simulink model "ASM_Traffic_V2X_Complete_Model_2"  (R2019a)
settings: Solver=ode1  StartTime=SIM.tstart.v  StopTime=Inf  FixedStep=SIM.StepSize.v  RelTol=1e-3
PostLoadFcn:
  | if any(exist('dsrtsu_mdlpostloadfcn', 'file') ~= 0), dsrtsu_mdlpostloadfcn('Execute', bdroot); end
  | try, asm_mdl_postloadfcn(bdroot, 'UpdateModel', 2200); catch, disp(lasterr); end,
undefined symbols (not defined in the file): _SensorPnts_1, _SensorPnts_13, _SensorPnts_17, _SensorPnts_21, _SensorPnts_25, _SensorPnts_29, _SensorPnts_33, _SensorPnts_37, _SensorPnts_41, _SensorPnts_45, _SensorPnts_49, _SensorPnts_5, _SensorPnts_53, _SensorPnts_57, _SensorPnts_9, _to_, CPT, G5A, ITS, MDL, rad, s_to_rpm, SIM
libraries: simulink x169, ASM_VehicleDynamics_lib x126, ASM_Traffic_lib x83, ASM_Utils_lib x49, mdbs x45, ASM_Environment_lib x17, dspindex x12, dsaV2xLibraryAux x10, dsmpblib x6, dsaV2xAsn1Library x4, dsaV2xLibrary x4, ASM_BrakeHydraulics_lib x4
(part 35 of 36)

== system ASM_Traffic_V2X_Complete_Model_2/IO/I//O_Subsystem/Bus Configuration (1) - Out/Simulated ECUs/DrivekitCAN/Drivekit/RX/PDUs/STEERING_TORQUE_COMMAND/steering_torque_command ==
  steering_torque_command : Inport
  ISignal Value : Subsystem
  _steering_torque_command_ : BusSelector  OutputSignals=ISignal Value
  wires:
  steering_torque_command/1 -> _steering_torque_command_/1  "steering_torque_command"
  _steering_torque_command_/1 -> ISignal Value/1(ISignal Value)  "<ISignal Value>"

== system ASM_Traffic_V2X_Complete_Model_2/IO/I//O_Subsystem/Bus Configuration (1) - Out/Simulated ECUs/DrivekitCAN/Drivekit/RX/PDUs/THROTTLE_COMMAND/throttle_command_magic ==
  throttle_command_magic : Inport
  ISignal Value : Subsystem
  _throttle_command_magic_ : BusSelector  OutputSignals=ISignal Value
  wires:
  throttle_command_magic/1 -> _throttle_command_magic_/1  "throttle_command_magic"
  _throttle_command_magic_/1 -> ISignal Value/1(ISignal Value)  "<ISignal Value>"

== system ASM_Traffic_V2X_Complete_Model_2/IO/I//O_Subsystem/Bus Configuration (1) - Out/Simulated ECUs/DrivekitCAN/Drivekit/RX/PDUs/THROTTLE_COMMAND/throttle_pedal_command ==
  throttle_pedal_command : Inport
  ISignal Value : Subsystem
  _throttle_pedal_command_ : BusSelector  OutputSignals=ISignal Value
  wires:
  throttle_pedal_command/1 -> _throttle_pedal_command_/1  "throttle_pedal_command"
  _throttle_pedal_command_/1 -> ISignal Value/1(ISignal Value)  "<ISignal Value>"

== system ASM_Traffic_V2X_Complete_Model_2/IO/I//O_Subsystem/Bus Configuration (1) - Out/Simulated ECUs/DrivekitCAN/Drivekit/RX/PDUs/THROTTLE_DISABLE/throttle_disable_magic ==
  throttle_disable_magic : Inport
  ISignal Value : Subsystem
  _throttle_disable_magic_ : BusSelector  OutputSignals=ISignal Value
  wires:
  throttle_disable_magic/1 -> _throttle_disable_magic_/1  "throttle_disable_magic"
  _throttle_disable_magic_/1 -> ISignal Value/1(ISignal Value)  "<ISignal Value>"

== system ASM_Traffic_V2X_Complete_Model_2/IO/I//O_Subsystem/Bus Configuration (1) - Out/Simulated ECUs/DrivekitCAN/Drivekit/RX/PDUs/THROTTLE_ENABLE/throttle_enable_magic ==
  throttle_enable_magic : Inport
  ISignal Value : Subsystem
  _throttle_enable_magic_ : BusSelector  OutputSignals=ISignal Value
  wires:
  throttle_enable_magic/1 -> _throttle_enable_magic_/1  "throttle_enable_magic"
  _throttle_enable_magic_/1 -> ISignal Value/1(ISignal Value)  "<ISignal Value>"

== system ASM_Traffic_V2X_Complete_Model_2/MDLUserInterface/MotionDeskInterface/MOTION_DESK_INTERFACE/Traffic_Animation/Sensors_Animation/Sensor_Points/Object_Sensor_2D_Points/Calc_Object_Sensor_2D_Points/Sensor_Points/ForIterator_Current ==
  dim_animation_point[] : Inport
  init_animation_point[] : Inport  Port=2
  num_sensor_rays[] : Inport  Port=3
  distance_sensor_out : Inport  Port=4
  angle_sensor_out : Inport  Port=5
  Add1 : Sum  Inputs=+-
  AnimationPoint_Idx : MultiPortSwitch  DataPortOrder=Zero-based contiguous  Inputs=2  zeroidx=on
  Assignment_Angle : Assignment  IndexOptions=Index vector (port)  Indices=1  OutputSizes=1
  Assignment_Distance : Assignment  IndexOptions=Index vector (port)  Indices=1  OutputSizes=1
  Calc_Output_Idx[] : Sum
  Calc_Saturated_Iteration_Idx : simulink/Discontinuities/Saturation Dynamic  OutMin=[]  OutMax=[]  OutDataTypeStr=Inherit: Same as second input  OutDataType=fixdt(1, 16)  OutScaling=2^-10  DoSatur=off
  Calc_Scaling_Step : Rounding  Operator=ceil
  Constant1 : Constant
  Constant2 : Constant
  Default_Idx : Constant
  Default_Value : Constant  Value=0
  Divide : Product  Inputs=*/
  For Iterator : ForIterator  ResetStates=reset  IterationSource=external  IterationLimit=36
  Iteration_Idx_LowBound : Constant
  Iteration_Idx_UpBound : MultiPortSwitch  DataPortOrder=Zero-based contiguous  Inputs=2  zeroidx=on
  Multiport Switch : MultiPortSwitch  DataPortOrder=Zero-based contiguous  Inputs=2  zeroidx=on
  Output_Idx : MultiPortSwitch  DataPortOrder=Zero-based contiguous  Inputs=2  zeroidx=on
  Point_Is_Unused : Constant  Value=0
  Product : Product
  Relational Operator : RelationalOperator  Operator=<=  OutDataTypeStr=boolean  RndMeth=Nearest
  Relational Operator1 : RelationalOperator  Operator=<  OutDataTypeStr=boolean  RndMeth=Nearest
  Relational Operator2 : RelationalOperator  Operator=<  OutDataTypeStr=boolean  RndMeth=Nearest
  Relational Operator3 : RelationalOperator  Operator=>  OutDataTypeStr=boolean  RndMeth=Nearest
  Saturate_to_sensor_output_dim : Saturate  UpperLimit=MDL.Traffic.Sensors.ObjectSensor2D_Calculation.Const_Sensor_Output_Dimension.v  LowerLimit=1
  Select_Angle : Selector  InputPortWidth=MDL.Traffic.Sensors.ObjectSensor2D_Calculation.Const_Sensor_Output_Dimension.v  IndexOptions=Starting index (port)  Indices=[1 3]  OutputSizes=1
  Select_Default_Angle : MultiPortSwitch  DataPortOrder=Zero-based contiguous  Inputs=2  zeroidx=on
  Select_Default_Distance : MultiPortSwitch  DataPortOrder=Zero-based contiguous  Inputs=2  zeroidx=on
  Select_Distance : Selector  InputPortWidth=MDL.Traffic.Sensors.ObjectSensor2D_Calculation.Const_Sensor_Output_Dimension.v  IndexOptions=Starting index (port)  Indices=[1 3]  OutputSizes=1
  distance_animation_point[m] : Outport  InitialOutput=0
  angle_animation_point[deg] : Outport  Port=2  InitialOutput=0
  flag_point_used[0|1] : Outport  Port=3  InitialOutput=0
  wires:
  Relational Operator3/1 -> flag_point_used[0|1]/1
  Select_Default_Angle/1 -> Assignment_Angle/2
  Default_Value/1 -> Select_Default_Angle/3, Select_Default_Distance/3
  Select_Default_Distance/1 -> Assignment_Distance/2
  num_sensor_rays[]/1 -> Saturate_to_sensor_output_dim/1
  dim_animation_point[]/1 -> Relational Operator/2, Divide/2, Relational Operator1/2, Iteration_Idx_UpBound/2, For Iterator/1
  Divide/1 -> Calc_Scaling_Step/1
  Calc_Saturated_Iteration_Idx/1 -> AnimationPoint_Idx/2, Add1/1
  Calc_Scaling_Step/1 -> Product/1
  Constant1/1 -> Add1/2
  Product/1 -> Calc_Output_Idx[]/1
  Constant2/1 -> Calc_Output_Idx[]/2
  Add1/1 -> Product/2
  Calc_Output_Idx[]/1 -> Relational Operator2/2, Output_Idx/2
  Default_Idx/1 -> Output_Idx/3, AnimationPoint_Idx/3
  Relational Operator2/1 -> Select_Default_Angle/1, Select_Default_Distance/1, Output_Idx/1, AnimationPoint_Idx/1
  Relational Operator1/1 -> Iteration_Idx_UpBound/1
  Iteration_Idx_UpBound/1 -> Calc_Saturated_Iteration_Idx/1
  Iteration_Idx_LowBound/1 -> Calc_Saturated_Iteration_Idx/3
  For Iterator/1 -> Calc_Saturated_Iteration_Idx/2
  AnimationPoint_Idx/1 -> Assignment_Distance/3, Assignment_Angle/3, Multiport Switch/3
  Multiport Switch/1 -> Select_Distance/2, Select_Angle/2
  Output_Idx/1 -> Multiport Switch/2
  Relational Operator/1 -> Multiport Switch/1
  Select_Angle/1 -> Select_Default_Angle/2
  Select_Distance/1 -> Select_Default_Distance/2
  distance_sensor_out/1 -> Select_Distance/1
  angle_sensor_out/1 -> Select_Angle/1
  Assignment_Angle/1 -> angle_animation_point[deg]/1
  Assignment_Distance/1 -> Relational Operator3/1, distance_animation_point[m]/1
  init_animation_point[]/1 -> Assignment_Angle/1, Assignment_Distance/1
  Saturate_to_sensor_output_dim/1 -> Relational Operator2/1, Divide/1, Relational Operator1/1, Iteration_Idx_UpBound/3, Relational Operator/1
  Point_Is_Unused/1 -> Relational Operator3/2

== system ASM_Traffic_V2X_Complete_Model_2/IO/I//O_Subsystem/Bus Configuration (1) - In/Simulated ECUs/DrivekitCAN/Drivekit/TX/PDUs/BRAKE_REPORT/PDU Features/PDU Cyclic Timing Control ==
  Const_BRAKE_REPORT Timing Control Offset : Constant  Value=0.02  OutDataTypeStr=double
  Const_BRAKE_REPORT Timing Control Period : Constant  Value=0.02  OutDataTypeStr=double
  _PDU Cyclic Timing Control_ : BusCreator  Inputs=2
  PDU Cyclic Timing Control : Outport
  wires:
  _PDU Cyclic Timing Control_/1 -> PDU Cyclic Timing Control/1  "PDU Cyclic Timing Control"
  Const_BRAKE_REPORT Timing Control Period/1 -> _PDU Cyclic Timing Control_/1  "BRAKE_REPORT Timing Control Period"
  Const_BRAKE_REPORT Timing Control Offset/1 -> _PDU Cyclic Timing Control_/2  "BRAKE_REPORT Timing Control Offset"

== system ASM_Traffic_V2X_Complete_Model_2/IO/I//O_Subsystem/Bus Configuration (1) - In/Simulated ECUs/DrivekitCAN/Drivekit/TX/PDUs/BRAKE_REPORT/brake_dtcs/ISignal Value ==
  Const_brake_dtcs Value : Constant  Value=0  OutDataTypeStr=uint8
  _ISignal Value_ : BusCreator  Inputs=1
  ISignal Value : Outport
  wires:
  _ISignal Value_/1 -> ISignal Value/1  "ISignal Value"
  Const_brake_dtcs Value/1 -> _ISignal Value_/1  "brake_dtcs Value"

== system ASM_Traffic_V2X_Complete_Model_2/IO/I//O_Subsystem/Bus Configuration (1) - In/Simulated ECUs/DrivekitCAN/Drivekit/TX/PDUs/BRAKE_REPORT/brake_operator_override/ISignal Value ==
  Const_brake_operator_override Value : Constant  Value=0  OutDataTypeStr=uint8
  _ISignal Value_ : BusCreator  Inputs=1
  ISignal Value : Outport
  wires:
  _ISignal Value_/1 -> ISignal Value/1  "ISignal Value"
  Const_brake_operator_override Value/1 -> _ISignal Value_/1  "brake_operator_override Value"

== system ASM_Traffic_V2X_Complete_Model_2/IO/I//O_Subsystem/Bus Configuration (1) - In/Simulated ECUs/DrivekitCAN/Drivekit/TX/PDUs/BRAKE_REPORT/brake_report_enabled/ISignal Value ==
  Const_brake_report_enabled Value : Constant  Value=0  OutDataTypeStr=uint8
  _ISignal Value_ : BusCreator  Inputs=1
  ISignal Value : Outport
  wires:
  _ISignal Value_/1 -> ISignal Value/1  "ISignal Value"
  Const_brake_report_enabled Value/1 -> _ISignal Value_/1  "brake_report_enabled Value"

== system ASM_Traffic_V2X_Complete_Model_2/IO/I//O_Subsystem/Bus Configuration (1) - In/Simulated ECUs/DrivekitCAN/Drivekit/TX/PDUs/BRAKE_REPORT/brake_report_magic/ISignal Value ==
  Const_brake_report_magic Value : Constant  Value=0  OutDataTypeStr=uint16
  _ISignal Value_ : BusCreator  Inputs=1
  ISignal Value : Outport
  wires:
  _ISignal Value_/1 -> ISignal Value/1  "ISignal Value"
  Const_brake_report_magic Value/1 -> _ISignal Value_/1  "brake_report_magic Value"

== system ASM_Traffic_V2X_Complete_Model_2/IO/I//O_Subsystem/Bus Configuration (1) - In/Simulated ECUs/DrivekitCAN/Drivekit/TX/PDUs/CHASSIS_CONTROL_REPORT/PDU Features/PDU Cyclic Timing Control ==
  Const_CHASSIS_CONTROL_REPORT Timing Control Offset : Constant  Value=10  OutDataTypeStr=double
  Const_CHASSIS_CONTROL_REPORT Timing Control Period : Constant  Value=10  OutDataTypeStr=double
  _PDU Cyclic Timing Control_ : BusCreator  Inputs=2
  PDU Cyclic Timing Control : Outport
  wires:
  _PDU Cyclic Timing Control_/1 -> PDU Cyclic Timing Control/1  "PDU Cyclic Timing Control"
  Const_CHASSIS_CONTROL_REPORT Timing Control Period/1 -> _PDU Cyclic Timing Control_/1  "CHASSIS_CONTROL_REPORT Timing Control Period"
  Const_CHASSIS_CONTROL_REPORT Timing Control Offset/1 -> _PDU Cyclic Timing Control_/2  "CHASSIS_CONTROL_REPORT Timing Control Offset"

== system ASM_Traffic_V2X_Complete_Model_2/IO/I//O_Subsystem/Bus Configuration (1) - In/Simulated ECUs/DrivekitCAN/Drivekit/TX/PDUs/CHASSIS_CONTROL_REPORT/front_wipers/ISignal Value ==
  Const_front_wipers Value : Constant  Value=0  OutDataTypeStr=uint8
  _ISignal Value_ : BusCreator  Inputs=1
  ISignal Value : Outport
  wires:
  _ISignal Value_/1 -> ISignal Value/1  "ISignal Value"
  Const_front_wipers Value/1 -> _ISignal Value_/1  "front_wipers Value"

== system ASM_Traffic_V2X_Complete_Model_2/IO/I//O_Subsystem/Bus Configuration (1) - In/Simulated ECUs/DrivekitCAN/Drivekit/TX/PDUs/CHASSIS_CONTROL_REPORT/headlamps/ISignal Value ==
  Const_headlamps Value : Constant  Value=0  OutDataTypeStr=uint8
  _ISignal Value_ : BusCreator  Inputs=1
  ISignal Value : Outport
  wires:
  _ISignal Value_/1 -> ISignal Value/1  "ISignal Value"
  Const_headlamps Value/1 -> _ISignal Value_/1  "headlamps Value"

== system ASM_Traffic_V2X_Complete_Model_2/IO/I//O_Subsystem/Bus Configuration (1) - In/Simulated ECUs/DrivekitCAN/Drivekit/TX/PDUs/CHASSIS_CONTROL_REPORT/horn/ISignal Value ==
  Const_horn Value : Constant  Value=0  OutDataTypeStr=uint8
  _ISignal Value_ : BusCreator  Inputs=1
  ISignal Value : Outport
  wires:
  _ISignal Value_/1 -> ISignal Value/1  "ISignal Value"
  Const_horn Value/1 -> _ISignal Value_/1  "horn Value"

== system ASM_Traffic_V2X_Complete_Model_2/IO/I//O_Subsystem/Bus Configuration (1) - In/Simulated ECUs/DrivekitCAN/Drivekit/TX/PDUs/CHASSIS_CONTROL_REPORT/left_signal/ISignal Value ==
  Const_left_signal Value : Constant  Value=0  OutDataTypeStr=uint8
  _ISignal Value_ : BusCreator  Inputs=1
  ISignal Value : Outport
  wires:
  _ISignal Value_/1 -> ISignal Value/1  "ISignal Value"
  Const_left_signal Value/1 -> _ISignal Value_/1  "left_signal Value"

== system ASM_Traffic_V2X_Complete_Model_2/IO/I//O_Subsystem/Bus Configuration (1) - In/Simulated ECUs/DrivekitCAN/Drivekit/TX/PDUs/CHASSIS_CONTROL_REPORT/rear_wiper/ISignal Value ==
  Const_rear_wiper Value : Constant  Value=0  OutDataTypeStr=uint8
  _ISignal Value_ : BusCreator  Inputs=1
  ISignal Value : Outport
  wires:
  _ISignal Value_/1 -> ISignal Value/1  "ISignal Value"
  Const_rear_wiper Value/1 -> _ISignal Value_/1  "rear_wiper Value"

== system ASM_Traffic_V2X_Complete_Model_2/IO/I//O_Subsystem/Bus Configuration (1) - In/Simulated ECUs/DrivekitCAN/Drivekit/TX/PDUs/CHASSIS_CONTROL_REPORT/right_signal/ISignal Value ==
  Const_right_signal Value : Constant  Value=0  OutDataTypeStr=uint8
  _ISignal Value_ : BusCreator  Inputs=1
  ISignal Value : Outport
  wires:
  _ISignal Value_/1 -> ISignal Value/1  "ISignal Value"
  Const_right_signal Value/1 -> _ISignal Value_/1  "right_signal Value"

== system ASM_Traffic_V2X_Complete_Model_2/IO/I//O_Subsystem/Bus Configuration (1) - In/Simulated ECUs/DrivekitCAN/Drivekit/TX/PDUs/CHASSIS_CONTROL_REPORT/vin_request/ISignal Value ==
  Const_vin_request Value : Constant  Value=0  OutDataTypeStr=uint8
  _ISignal Value_ : BusCreator  Inputs=1
  ISignal Value : Outport
  wires:
  _ISignal Value_/1 -> ISignal Value/1  "ISignal Value"
  Const_vin_request Value/1 -> _ISignal Value_/1  "vin_request Value"

== system ASM_Traffic_V2X_Complete_Model_2/IO/I//O_Subsystem/Bus Configuration (1) - In/Simulated ECUs/DrivekitCAN/Drivekit/TX/PDUs/ESP12/CYL_PRES/ISignal Value ==
  Const_CYL_PRES Value : Constant  Value=0  OutDataTypeStr=double
  _ISignal Value_ : BusCreator  Inputs=1
  ISignal Value : Outport
  wires:
  _ISignal Value_/1 -> ISignal Value/1  "ISignal Value"
  Const_CYL_PRES Value/1 -> _ISignal Value_/1  "CYL_PRES Value"

== system ASM_Traffic_V2X_Complete_Model_2/IO/I//O_Subsystem/Bus Configuration (1) - In/Simulated ECUs/DrivekitCAN/Drivekit/TX/PDUs/ESP12/CYL_PRESS_DIAG/ISignal Value ==
  Const_CYL_PRESS_DIAG Value : Constant  Value=0  OutDataTypeStr=uint8
  _ISignal Value_ : BusCreator  Inputs=1
  ISignal Value : Outport
  wires:
  _ISignal Value_/1 -> ISignal Value/1  "ISignal Value"
  Const_CYL_PRESS_DIAG Value/1 -> _ISignal Value_/1  "CYL_PRESS_DIAG Value"

== system ASM_Traffic_V2X_Complete_Model_2/IO/I//O_Subsystem/Bus Configuration (1) - In/Simulated ECUs/DrivekitCAN/Drivekit/TX/PDUs/ESP12/CYL_PRES_STAT/ISignal Value ==
  Const_CYL_PRES_STAT Value : Constant  Value=0  OutDataTypeStr=uint8
  _ISignal Value_ : BusCreator  Inputs=1
  ISignal Value : Outport
  wires:
  _ISignal Value_/1 -> ISignal Value/1  "ISignal Value"
  Const_CYL_PRES_STAT Value/1 -> _ISignal Value_/1  "CYL_PRES_STAT Value"

== system ASM_Traffic_V2X_Complete_Model_2/IO/I//O_Subsystem/Bus Configuration (1) - In/Simulated ECUs/DrivekitCAN/Drivekit/TX/PDUs/ESP12/ESP12_AliveCounter/ISignal Value ==
  Const_ESP12_AliveCounter Value : Constant  Value=0  OutDataTypeStr=uint8
  _ISignal Value_ : BusCreator  Inputs=1
  ISignal Value : Outport
  wires:
  _ISignal Value_/1 -> ISignal Value/1  "ISignal Value"
  Const_ESP12_AliveCounter Value/1 -> _ISignal Value_/1  "ESP12_AliveCounter Value"

== system ASM_Traffic_V2X_Complete_Model_2/IO/I//O_Subsystem/Bus Configuration (1) - In/Simulated ECUs/DrivekitCAN/Drivekit/TX/PDUs/ESP12/ESP12_Checksum/ISignal Value ==
  Const_ESP12_Checksum Value : Constant  Value=0  OutDataTypeStr=uint8
  _ISignal Value_ : BusCreator  Inputs=1
  ISignal Value : Outport
  wires:
  _ISignal Value_/1 -> ISignal Value/1  "ISignal Value"
  Const_ESP12_Checksum Value/1 -> _ISignal Value_/1  "ESP12_Checksum Value"

== system ASM_Traffic_V2X_Complete_Model_2/IO/I//O_Subsystem/Bus Configuration (1) - In/Simulated ECUs/DrivekitCAN/Drivekit/TX/PDUs/ESP12/LAT_ACCEL/ISignal Value ==
  Const_LAT_ACCEL Value : Constant  Value=-10.23  OutDataTypeStr=double
  _ISignal Value_ : BusCreator  Inputs=1
  ISignal Value : Outport
  wires:
  _ISignal Value_/1 -> ISignal Value/1  "ISignal Value"
  Const_LAT_ACCEL Value/1 -> _ISignal Value_/1  "LAT_ACCEL Value"

== system ASM_Traffic_V2X_Complete_Model_2/IO/I//O_Subsystem/Bus Configuration (1) - In/Simulated ECUs/DrivekitCAN/Drivekit/TX/PDUs/ESP12/LAT_ACCEL_DIAG/ISignal Value ==
  Const_LAT_ACCEL_DIAG Value : Constant  Value=0  OutDataTypeStr=uint8
  _ISignal Value_ : BusCreator  Inputs=1
  ISignal Value : Outport
  wires:
  _ISignal Value_/1 -> ISignal Value/1  "ISignal Value"
  Const_LAT_ACCEL_DIAG Value/1 -> _ISignal Value_/1  "LAT_ACCEL_DIAG Value"

== system ASM_Traffic_V2X_Complete_Model_2/IO/I//O_Subsystem/Bus Configuration (1) - In/Simulated ECUs/DrivekitCAN/Drivekit/TX/PDUs/ESP12/LAT_ACCEL_STAT/ISignal Value ==
  Const_LAT_ACCEL_STAT Value : Constant  Value=0  OutDataTypeStr=uint8
  _ISignal Value_ : BusCreator  Inputs=1
  ISignal Value : Outport
  wires:
  _ISignal Value_/1 -> ISignal Value/1  "ISignal Value"
  Const_LAT_ACCEL_STAT Value/1 -> _ISignal Value_/1  "LAT_ACCEL_STAT Value"

== system ASM_Traffic_V2X_Complete_Model_2/IO/I//O_Subsystem/Bus Configuration (1) - In/Simulated ECUs/DrivekitCAN/Drivekit/TX/PDUs/ESP12/LONG_ACCEL/ISignal Value ==
  Const_LONG_ACCEL Value : Constant  Value=-10.23  OutDataTypeStr=double
  _ISignal Value_ : BusCreator  Inputs=1
  ISignal Value : Outport
  wires:
  _ISignal Value_/1 -> ISignal Value/1  "ISignal Value"
  Const_LONG_ACCEL Value/1 -> _ISignal Value_/1  "LONG_ACCEL Value"

== system ASM_Traffic_V2X_Complete_Model_2/IO/I//O_Subsystem/Bus Configuration (1) - In/Simulated ECUs/DrivekitCAN/Drivekit/TX/PDUs/ESP12/LONG_ACCEL_DIAG/ISignal Value ==
  Const_LONG_ACCEL_DIAG Value : Constant  Value=0  OutDataTypeStr=uint8
  _ISignal Value_ : BusCreator  Inputs=1
  ISignal Value : Outport
  wires:
  _ISignal Value_/1 -> ISignal Value/1  "ISignal Value"
  Const_LONG_ACCEL_DIAG Value/1 -> _ISignal Value_/1  "LONG_ACCEL_DIAG Value"

== system ASM_Traffic_V2X_Complete_Model_2/IO/I//O_Subsystem/Bus Configuration (1) - In/Simulated ECUs/DrivekitCAN/Drivekit/TX/PDUs/ESP12/LONG_ACCEL_STAT/ISignal Value ==
  Const_LONG_ACCEL_STAT Value : Constant  Value=0  OutDataTypeStr=uint8
  _ISignal Value_ : BusCreator  Inputs=1
  ISignal Value : Outport
  wires:
  _ISignal Value_/1 -> ISignal Value/1  "ISignal Value"
  Const_LONG_ACCEL_STAT Value/1 -> _ISignal Value_/1  "LONG_ACCEL_STAT Value"

== system ASM_Traffic_V2X_Complete_Model_2/IO/I//O_Subsystem/Bus Configuration (1) - In/Simulated ECUs/DrivekitCAN/Drivekit/TX/PDUs/ESP12/PDU Features/PDU Cyclic Timing Control ==
  Const_ESP12 Timing Control Offset : Constant  Value=10  OutDataTypeStr=double
  Const_ESP12 Timing Control Period : Constant  Value=10  OutDataTypeStr=double
  _PDU Cyclic Timing Control_ : BusCreator  Inputs=2
  PDU Cyclic Timing Control : Outport
  wires:
  _PDU Cyclic Timing Control_/1 -> PDU Cyclic Timing Control/1  "PDU Cyclic Timing Control"
  Const_ESP12 Timing Control Period/1 -> _PDU Cyclic Timing Control_/1  "ESP12 Timing Control Period"
  Const_ESP12 Timing Control Offset/1 -> _PDU Cyclic Timing Control_/2  "ESP12 Timing Control Offset"

== system ASM_Traffic_V2X_Complete_Model_2/IO/I//O_Subsystem/Bus Configuration (1) - In/Simulated ECUs/DrivekitCAN/Drivekit/TX/PDUs/ESP12/YAW_RATE/ISignal Value ==
  Const_YAW_RATE Value : Constant  Value=-40.95  OutDataTypeStr=double
  _ISignal Value_ : BusCreator  Inputs=1
  ISignal Value : Outport
  wires:
  _ISignal Value_/1 -> ISignal Value/1  "ISignal Value"
  Const_YAW_RATE Value/1 -> _ISignal Value_/1  "YAW_RATE Value"

== system ASM_Traffic_V2X_Complete_Model_2/IO/I//O_Subsystem/Bus Configuration (1) - In/Simulated ECUs/DrivekitCAN/Drivekit/TX/PDUs/ESP12/YAW_RATE_DIAG/ISignal Value ==
  Const_YAW_RATE_DIAG Value : Constant  Value=0  OutDataTypeStr=uint8
  _ISignal Value_ : BusCreator  Inputs=1
  ISignal Value : Outport
  wires:
  _ISignal Value_/1 -> ISignal Value/1  "ISignal Value"
  Const_YAW_RATE_DIAG Value/1 -> _ISignal Value_/1  "YAW_RATE_DIAG Value"

== system ASM_Traffic_V2X_Complete_Model_2/IO/I//O_Subsystem/Bus Configuration (1) - In/Simulated ECUs/DrivekitCAN/Drivekit/TX/PDUs/ESP12/YAW_RATE_STAT/ISignal Value ==
  Const_YAW_RATE_STAT Value : Constant  Value=0  OutDataTypeStr=uint8
  _ISignal Value_ : BusCreator  Inputs=1
  ISignal Value : Outport
  wires:
  _ISignal Value_/1 -> ISignal Value/1  "ISignal Value"
  Const_YAW_RATE_STAT Value/1 -> _ISignal Value_/1  "YAW_RATE_STAT Value"

== system ASM_Traffic_V2X_Complete_Model_2/IO/I//O_Subsystem/Bus Configuration (1) - In/Simulated ECUs/DrivekitCAN/Drivekit/TX/PDUs/FAULT_REPORT/PDU Features/PDU Cyclic Timing Control ==
  Const_FAULT_REPORT Timing Control Offset : Constant  Value=10  OutDataTypeStr=double
  Const_FAULT_REPORT Timing Control Period : Constant  Value=10  OutDataTypeStr=double
  _PDU Cyclic Timing Control_ : BusCreator  Inputs=2
  PDU Cyclic Timing Control : Outport
  wires:
  _PDU Cyclic Timing Control_/1 -> PDU Cyclic Timing Control/1  "PDU Cyclic Timing Control"
  Const_FAULT_REPORT Timing Control Period/1 -> _PDU Cyclic Timing Control_/1  "FAULT_REPORT Timing Control Period"
  Const_FAULT_REPORT Timing Control Offset/1 -> _PDU Cyclic Timing Control_/2  "FAULT_REPORT Timing Control Offset"

== system ASM_Traffic_V2X_Complete_Model_2/IO/I//O_Subsystem/Bus Configuration (1) - In/Simulated ECUs/DrivekitCAN/Drivekit/TX/PDUs/FAULT_REPORT/fault_dtcs/ISignal Value ==
  Const_fault_dtcs Value : Constant  Value=0  OutDataTypeStr=uint8
  _ISignal Value_ : BusCreator  Inputs=1
  ISignal Value : Outport
  wires:
  _ISignal Value_/1 -> ISignal Value/1  "ISignal Value"
  Const_fault_dtcs Value/1 -> _ISignal Value_/1  "fault_dtcs Value"

== system ASM_Traffic_V2X_Complete_Model_2/IO/I//O_Subsystem/Bus Configuration (1) - In/Simulated ECUs/DrivekitCAN/Drivekit/TX/PDUs/FAULT_REPORT/fault_origin_id/ISignal Value ==
  Const_fault_origin_id Value : Constant  Value=0  OutDataTypeStr=uint32
  _ISignal Value_ : BusCreator  Inputs=1
  ISignal Value : Outport
  wires:
  _ISignal Value_/1 -> ISignal Value/1  "ISignal Value"
  Const_fault_origin_id Value/1 -> _ISignal Value_/1  "fault_origin_id Value"

== system ASM_Traffic_V2X_Complete_Model_2/IO/I//O_Subsystem/Bus Configuration (1) - In/Simulated ECUs/DrivekitCAN/Drivekit/TX/PDUs/FAULT_REPORT/fault_report_magic/ISignal Value ==
  Const_fault_report_magic Value : Constant  Value=0  OutDataTypeStr=uint16
  _ISignal Value_ : BusCreator  Inputs=1
  ISignal Value : Outport
  wires:
  _ISignal Value_/1 -> ISignal Value/1  "ISignal Value"
  Const_fault_report_magic Value/1 -> _ISignal Value_/1  "fault_report_magic Value"

== system ASM_Traffic_V2X_Complete_Model_2/IO/I//O_Subsystem/Bus Configuration (1) - In/Simulated ECUs/DrivekitCAN/Drivekit/TX/PDUs/GPS_HEADING/Heading/ISignal Value ==
  Input : Inport
  Const_Heading Value : Constant  Value=0  OutDataTypeStr=double
  Data Type Conversion : DataTypeConversion
  Gain : Gain
  Terminator : Terminator
  _ISignal Value_ : BusCreator  Inputs=1
  ISignal Value : Outport
  wires:
  _ISignal Value_/1 -> ISignal Value/1  "ISignal Value"
  Const_Heading Value/1 -> Terminator/1  "Heading Value"
  Input/1 -> Gain/1  "Heading Value"
  Gain/1 -> Data Type Conversion/1  "Heading Value"
  Data Type Conversion/1 -> _ISignal Value_/1  "Heading Value"

== system ASM_Traffic_V2X_Complete_Model_2/IO/I//O_Subsystem/Bus Configuration (1) - In/Simulated ECUs/DrivekitCAN/Drivekit/TX/PDUs/GPS_HEADING/PDU Features/PDU Cyclic Timing Control ==
  Const_GPS_HEADING Timing Control Offset : Constant  OutDataTypeStr=double
  Const_GPS_HEADING Timing Control Period : Constant  OutDataTypeStr=double
  _PDU Cyclic Timing Control_ : BusCreator  Inputs=2
  PDU Cyclic Timing Control : Outport
  wires:
  _PDU Cyclic Timing Control_/1 -> PDU Cyclic Timing Control/1  "PDU Cyclic Timing Control"
  Const_GPS_HEADING Timing Control Period/1 -> _PDU Cyclic Timing Control_/1  "GPS_HEADING Timing Control Period"
  Const_GPS_HEADING Timing Control Offset/1 -> _PDU Cyclic Timing Control_/2  "GPS_HEADING Timing Control Offset"

== system ASM_Traffic_V2X_Complete_Model_2/IO/I//O_Subsystem/Bus Configuration (1) - In/Simulated ECUs/DrivekitCAN/Drivekit/TX/PDUs/GPS_LAT/Lat/ISignal Value ==
  Input : Inport
  Const_Lat Value : Constant  Value=0  OutDataTypeStr=double
  Gain : Gain
  Terminator : Terminator
  _ISignal Value_ : BusCreator  Inputs=1
  ISignal Value : Outport
  wires:
  _ISignal Value_/1 -> ISignal Value/1  "ISignal Value"
  Const_Lat Value/1 -> Terminator/1  "Lat Value"
  Input/1 -> Gain/1  "Lat Value"
  Gain/1 -> _ISignal Value_/1  "Lat Value"

== system ASM_Traffic_V2X_Complete_Model_2/IO/I//O_Subsystem/Bus Configuration (1) - In/Simulated ECUs/DrivekitCAN/Drivekit/TX/PDUs/GPS_LAT/PDU Features/PDU Cyclic Timing Control ==
  Const_GPS_LAT Timing Control Offset : Constant  Value=0.02  OutDataTypeStr=double
  Const_GPS_LAT Timing Control Period : Constant  Value=0.02  OutDataTypeStr=double
  _PDU Cyclic Timing Control_ : BusCreator  Inputs=2
  PDU Cyclic Timing Control : Outport
  wires:
  _PDU Cyclic Timing Control_/1 -> PDU Cyclic Timing Control/1  "PDU Cyclic Timing Control"
  Const_GPS_LAT Timing Control Period/1 -> _PDU Cyclic Timing Control_/1  "GPS_LAT Timing Control Period"
  Const_GPS_LAT Timing Control Offset/1 -> _PDU Cyclic Timing Control_/2  "GPS_LAT Timing Control Offset"

== system ASM_Traffic_V2X_Complete_Model_2/IO/I//O_Subsystem/Bus Configuration (1) - In/Simulated ECUs/DrivekitCAN/Drivekit/TX/PDUs/GPS_LONG/Long/ISignal Value ==
  Input : Inport
  Const_Long Value : Constant  Value=0  OutDataTypeStr=double
  Gain : Gain
  Terminator : Terminator
  _ISignal Value_ : BusCreator  Inputs=1
  ISignal Value : Outport
  wires:
  _ISignal Value_/1 -> ISignal Value/1  "ISignal Value"
  Const_Long Value/1 -> Terminator/1  "Long Value"
  Input/1 -> Gain/1  "Long Value"
  Gain/1 -> _ISignal Value_/1  "Long Value"

== system ASM_Traffic_V2X_Complete_Model_2/IO/I//O_Subsystem/Bus Configuration (1) - In/Simulated ECUs/DrivekitCAN/Drivekit/TX/PDUs/GPS_LONG/PDU Features/PDU Cyclic Timing Control ==
  Const_GPS_LONG Timing Control Offset : Constant  Value=0.02  OutDataTypeStr=double
  Const_GPS_LONG Timing Control Period : Constant  Value=0.02  OutDataTypeStr=double
  _PDU Cyclic Timing Control_ : BusCreator  Inputs=2
  PDU Cyclic Timing Control : Outport
  wires:
  _PDU Cyclic Timing Control_/1 -> PDU Cyclic Timing Control/1  "PDU Cyclic Timing Control"
  Const_GPS_LONG Timing Control Period/1 -> _PDU Cyclic Timing Control_/1  "GPS_LONG Timing Control Period"
  Const_GPS_LONG Timing Control Offset/1 -> _PDU Cyclic Timing Control_/2  "GPS_LONG Timing Control Offset"

== system ASM_Traffic_V2X_Complete_Model_2/IO/I//O_Subsystem/Bus Configuration (1) - In/Simulated ECUs/DrivekitCAN/Drivekit/TX/PDUs/LANE_REPORT/PDU Features/PDU Cyclic Timing Control ==
  Const_LANE_REPORT Timing Control Offset : Constant  Value=0.02  OutDataTypeStr=double
  Const_LANE_REPORT Timing Control Period : Constant  Value=0.02  OutDataTypeStr=double
  _PDU Cyclic Timing Control_ : BusCreator  Inputs=2
  PDU Cyclic Timing Control : Outport
  wires:
  _PDU Cyclic Timing Control_/1 -> PDU Cyclic Timing Control/1  "PDU Cyclic Timing Control"
  Const_LANE_REPORT Timing Control Period/1 -> _PDU Cyclic Timing Control_/1  "LANE_REPORT Timing Control Period"
  Const_LANE_REPORT Timing Control Offset/1 -> _PDU Cyclic Timing Control_/2  "LANE_REPORT Timing Control Offset"

== system ASM_Traffic_V2X_Complete_Model_2/IO/I//O_Subsystem/Bus Configuration (1) - In/Simulated ECUs/DrivekitCAN/Drivekit/TX/PDUs/LANE_REPORT/lane_number/ISignal Value ==
  Input : Inport
  Const_lane_number Value : Constant  Value=0  OutDataTypeStr=single
  Data Type Conversion : DataTypeConversion
  Gain : Gain
  Terminator : Terminator
  _ISignal Value_ : BusCreator  Inputs=1
  ISignal Value : Outport
  wires:
  _ISignal Value_/1 -> ISignal Value/1  "ISignal Value"
  Const_lane_number Value/1 -> Terminator/1  "lane_number Value"
  Input/1 -> Gain/1
  Gain/1 -> Data Type Conversion/1  "lane_number Value"
  Data Type Conversion/1 -> _ISignal Value_/1  "lane_number Value"

== system ASM_Traffic_V2X_Complete_Model_2/IO/I//O_Subsystem/Bus Configuration (1) - In/Simulated ECUs/DrivekitCAN/Drivekit/TX/PDUs/LANE_REPORT/left_marker_distance/ISignal Value ==
  Input : Inport
  Const_left_marker_distance Value : Constant  Value=0  OutDataTypeStr=single
  Data Type Conversion : DataTypeConversion
  Gain : Gain
  Terminator : Terminator
  _ISignal Value_ : BusCreator  Inputs=1
  ISignal Value : Outport
  wires:
  _ISignal Value_/1 -> ISignal Value/1  "ISignal Value"
  Const_left_marker_distance Value/1 -> Terminator/1  "left_marker_distance Value"
  Input/1 -> Gain/1
  Gain/1 -> Data Type Conversion/1  "left_marker_distance Value"
  Data Type Conversion/1 -> _ISignal Value_/1  "left_marker_distance Value"

== system ASM_Traffic_V2X_Complete_Model_2/IO/I//O_Subsystem/Bus Configuration (1) - In/Simulated ECUs/DrivekitCAN/Drivekit/TX/PDUs/LANE_REPORT/right_marker_distance/ISignal Value ==
  Input : Inport
  Const_right_marker_distance Value : Constant  Value=0  OutDataTypeStr=single
  Data Type Conversion : DataTypeConversion
  Gain : Gain
  Terminator : Terminator
  _ISignal Value_ : BusCreator  Inputs=1
  ISignal Value : Outport
  wires:
  _ISignal Value_/1 -> ISignal Value/1  "ISignal Value"
  Const_right_marker_distance Value/1 -> Terminator/1  "right_marker_distance Value"
  Input/1 -> Gain/1
  Gain/1 -> Data Type Conversion/1  "right_marker_distance Value"
  Data Type Conversion/1 -> _ISignal Value_/1  "right_marker_distance Value"

== system ASM_Traffic_V2X_Complete_Model_2/IO/I//O_Subsystem/Bus Configuration (1) - In/Simulated ECUs/DrivekitCAN/Drivekit/TX/PDUs/SAS11/PDU Features/PDU Cyclic Timing Control ==
  Const_SAS11 Timing Control Offset : Constant  Value=0.02  OutDataTypeStr=double
  Const_SAS11 Timing Control Period : Constant  Value=0.02  OutDataTypeStr=double
  _PDU Cyclic Timing Control_ : BusCreator  Inputs=2
  PDU Cyclic Timing Control : Outport
  wires:
  _PDU Cyclic Timing Control_/1 -> PDU Cyclic Timing Control/1  "PDU Cyclic Timing Control"
  Const_SAS11 Timing Control Period/1 -> _PDU Cyclic Timing Control_/1  "SAS11 Timing Control Period"
  Const_SAS11 Timing Control Offset/1 -> _PDU Cyclic Timing Control_/2  "SAS11 Timing Control Offset"

== system ASM_Traffic_V2X_Complete_Model_2/IO/I//O_Subsystem/Bus Configuration (1) - In/Simulated ECUs/DrivekitCAN/Drivekit/TX/PDUs/SAS11/SAS_Angle/ISignal Value ==
  Input : Inport
  Const_SAS_Angle Value : Constant  Value=0  OutDataTypeStr=double
  Terminator : Terminator
  _ISignal Value_ : BusCreator  Inputs=1
  ISignal Value : Outport
  wires:
  _ISignal Value_/1 -> ISignal Value/1  "ISignal Value"
  Const_SAS_Angle Value/1 -> Terminator/1  "SAS_Angle Value"
  Input/1 -> _ISignal Value_/1  "SAS_Angle Value"

== system ASM_Traffic_V2X_Complete_Model_2/IO/I//O_Subsystem/Bus Configuration (1) - In/Simulated ECUs/DrivekitCAN/Drivekit/TX/PDUs/SAS11/SAS_CheckSum/ISignal Value ==
  Const_SAS_CheckSum Value : Constant  Value=0  OutDataTypeStr=uint8
  _ISignal Value_ : BusCreator  Inputs=1
  ISignal Value : Outport
  wires:
  _ISignal Value_/1 -> ISignal Value/1  "ISignal Value"
  Const_SAS_CheckSum Value/1 -> _ISignal Value_/1  "SAS_CheckSum Value"

== system ASM_Traffic_V2X_Complete_Model_2/IO/I//O_Subsystem/Bus Configuration (1) - In/Simulated ECUs/DrivekitCAN/Drivekit/TX/PDUs/SAS11/SAS_MsgCount/ISignal Value ==
  Const_SAS_MsgCount Value : Constant  Value=0  OutDataTypeStr=uint8
  _ISignal Value_ : BusCreator  Inputs=1
  ISignal Value : Outport
  wires:
  _ISignal Value_/1 -> ISignal Value/1  "ISignal Value"
  Const_SAS_MsgCount Value/1 -> _ISignal Value_/1  "SAS_MsgCount Value"

== system ASM_Traffic_V2X_Complete_Model_2/IO/I//O_Subsystem/Bus Configuration (1) - In/Simulated ECUs/DrivekitCAN/Drivekit/TX/PDUs/SAS11/SAS_Speed/ISignal Value ==
  Const_SAS_Speed Value : Constant  Value=0  OutDataTypeStr=uint16
  _ISignal Value_ : BusCreator  Inputs=1
  ISignal Value : Outport
  wires:
  _ISignal Value_/1 -> ISignal Value/1  "ISignal Value"
  Const_SAS_Speed Value/1 -> _ISignal Value_/1  "SAS_Speed Value"

== system ASM_Traffic_V2X_Complete_Model_2/IO/I//O_Subsystem/Bus Configuration (1) - In/Simulated ECUs/DrivekitCAN/Drivekit/TX/PDUs/SAS11/SAS_Stat/ISignal Value ==
  Const_SAS_Stat Value : Constant  Value=0  OutDataTypeStr=uint8
  _ISignal Value_ : BusCreator  Inputs=1
  ISignal Value : Outport
  wires:
  _ISignal Value_/1 -> ISignal Value/1  "ISignal Value"
  Const_SAS_Stat Value/1 -> _ISignal Value_/1  "SAS_Stat Value"

== system ASM_Traffic_V2X_Complete_Model_2/IO/I//O_Subsystem/Bus Configuration (1) - In/Simulated ECUs/DrivekitCAN/Drivekit/TX/PDUs/STEERING_ANGLE_REPORT/PDU Features/PDU Cyclic Timing Control ==
  Const_STEERING_ANGLE_REPORT Timing Control Offset : Constant  Value=0.02  OutDataTypeStr=double
  Const_STEERING_ANGLE_REPORT Timing Control Period : Constant  Value=0.02  OutDataTypeStr=double
  _PDU Cyclic Timing Control_ : BusCreator  Inputs=2
  PDU Cyclic Timing Control : Outport
  wires:
  _PDU Cyclic Timing Control_/1 -> PDU Cyclic Timing Control/1  "PDU Cyclic Timing Control"
  Const_STEERING_ANGLE_REPORT Timing Control Period/1 -> _PDU Cyclic Timing Control_/1  "STEERING_ANGLE_REPORT Timing Control Period"
  Const_STEERING_ANGLE_REPORT Timing Control Offset/1 -> _PDU Cyclic Timing Control_/2  "STEERING_ANGLE_REPORT Timing Control Offset"

== system ASM_Traffic_V2X_Complete_Model_2/IO/I//O_Subsystem/Bus Configuration (1) - In/Simulated ECUs/DrivekitCAN/Drivekit/TX/PDUs/STEERING_ANGLE_REPORT/steering_angle_report_errors/ISignal Value ==
  Const_steering_angle_report_errors Value : Constant  Value=0  OutDataTypeStr=uint8
  _ISignal Value_ : BusCreator  Inputs=1
  ISignal Value : Outport
  wires:
  _ISignal Value_/1 -> ISignal Value/1  "ISignal Value"
  Const_steering_angle_report_errors Value/1 -> _ISignal Value_/1  "steering_angle_report_errors Value"

== system ASM_Traffic_V2X_Complete_Model_2/IO/I//O_Subsystem/Bus Configuration (1) - In/Simulated ECUs/DrivekitCAN/Drivekit/TX/PDUs/STEERING_ANGLE_REPORT/steering_angle_report_flags/ISignal Value ==
  Const_steering_angle_report_flags Value : Constant  Value=0  OutDataTypeStr=uint8
  _ISignal Value_ : BusCreator  Inputs=1
  ISignal Value : Outport
  wires:
  _ISignal Value_/1 -> ISignal Value/1  "ISignal Value"
  Const_steering_angle_report_flags Value/1 -> _ISignal Value_/1  "steering_angle_report_flags Value"

== system ASM_Traffic_V2X_Complete_Model_2/IO/I//O_Subsystem/Bus Configuration (1) - In/Simulated ECUs/DrivekitCAN/Drivekit/TX/PDUs/STEERING_REPORT/PDU Features/PDU Cyclic Timing Control ==
  Const_STEERING_REPORT Timing Control Offset : Constant  Value=0.02  OutDataTypeStr=double
  Const_STEERING_REPORT Timing Control Period : Constant  Value=0.02  OutDataTypeStr=double
  _PDU Cyclic Timing Control_ : BusCreator  Inputs=2
  PDU Cyclic Timing Control : Outport
  wires:
  _PDU Cyclic Timing Control_/1 -> PDU Cyclic Timing Control/1  "PDU Cyclic Timing Control"
  Const_STEERING_REPORT Timing Control Period/1 -> _PDU Cyclic Timing Control_/1  "STEERING_REPORT Timing Control Period"
  Const_STEERING_REPORT Timing Control Offset/1 -> _PDU Cyclic Timing Control_/2  "STEERING_REPORT Timing Control Offset"

== system ASM_Traffic_V2X_Complete_Model_2/IO/I//O_Subsystem/Bus Configuration (1) - In/Simulated ECUs/DrivekitCAN/Drivekit/TX/PDUs/STEERING_REPORT/steering_dtcs/ISignal Value ==
  Const_steering_dtcs Value : Constant  Value=0  OutDataTypeStr=uint8
  _ISignal Value_ : BusCreator  Inputs=1
  ISignal Value : Outport
  wires:
  _ISignal Value_/1 -> ISignal Value/1  "ISignal Value"
  Const_steering_dtcs Value/1 -> _ISignal Value_/1  "steering_dtcs Value"

== system ASM_Traffic_V2X_Complete_Model_2/IO/I//O_Subsystem/Bus Configuration (1) - In/Simulated ECUs/DrivekitCAN/Drivekit/TX/PDUs/STEERING_REPORT/steering_operator_override/ISignal Value ==
  Const_steering_operator_override Value : Constant  Value=0  OutDataTypeStr=uint8
  _ISignal Value_ : BusCreator  Inputs=1
  ISignal Value : Outport
  wires:
  _ISignal Value_/1 -> ISignal Value/1  "ISignal Value"
  Const_steering_operator_override Value/1 -> _ISignal Value_/1  "steering_operator_override Value"

== system ASM_Traffic_V2X_Complete_Model_2/IO/I//O_Subsystem/Bus Configuration (1) - In/Simulated ECUs/DrivekitCAN/Drivekit/TX/PDUs/STEERING_REPORT/steering_report_enabled/ISignal Value ==
  Const_steering_report_enabled Value : Constant  Value=0  OutDataTypeStr=uint8
  _ISignal Value_ : BusCreator  Inputs=1
  ISignal Value : Outport
  wires:
  _ISignal Value_/1 -> ISignal Value/1  "ISignal Value"
  Const_steering_report_enabled Value/1 -> _ISignal Value_/1  "steering_report_enabled Value"

== system ASM_Traffic_V2X_Complete_Model_2/IO/I//O_Subsystem/Bus Configuration (1) - In/Simulated ECUs/DrivekitCAN/Drivekit/TX/PDUs/STEERING_REPORT/steering_report_magic/ISignal Value ==
  Const_steering_report_magic Value : Constant  Value=0  OutDataTypeStr=uint16
  _ISignal Value_ : BusCreator  Inputs=1
  ISignal Value : Outport
  wires:
  _ISignal Value_/1 -> ISignal Value/1  "ISignal Value"
  Const_steering_report_magic Value/1 -> _ISignal Value_/1  "steering_report_magic Value"

== system ASM_Traffic_V2X_Complete_Model_2/IO/I//O_Subsystem/Bus Configuration (1) - In/Simulated ECUs/DrivekitCAN/Drivekit/TX/PDUs/THROTTLE_REPORT/PDU Features/PDU Cyclic Timing Control ==
  Const_THROTTLE_REPORT Timing Control Offset : Constant  Value=0.02  OutDataTypeStr=double
  Const_THROTTLE_REPORT Timing Control Period : Constant  Value=0.02  OutDataTypeStr=double
  _PDU Cyclic Timing Control_ : BusCreator  Inputs=2
  PDU Cyclic Timing Control : Outport
  wires:
  _PDU Cyclic Timing Control_/1 -> PDU Cyclic Timing Control/1  "PDU Cyclic Timing Control"
  Const_THROTTLE_REPORT Timing Control Period/1 -> _PDU Cyclic Timing Control_/1  "THROTTLE_REPORT Timing Control Period"
  Const_THROTTLE_REPORT Timing Control Offset/1 -> _PDU Cyclic Timing Control_/2  "THROTTLE_REPORT Timing Control Offset"

== system ASM_Traffic_V2X_Complete_Model_2/IO/I//O_Subsystem/Bus Configuration (1) - In/Simulated ECUs/DrivekitCAN/Drivekit/TX/PDUs/THROTTLE_REPORT/throttle_dtcs/ISignal Value ==
  Const_throttle_dtcs Value : Constant  Value=0  OutDataTypeStr=uint8
  _ISignal Value_ : BusCreator  Inputs=1
  ISignal Value : Outport
  wires:
  _ISignal Value_/1 -> ISignal Value/1  "ISignal Value"
  Const_throttle_dtcs Value/1 -> _ISignal Value_/1  "throttle_dtcs Value"

== system ASM_Traffic_V2X_Complete_Model_2/IO/I//O_Subsystem/Bus Configuration (1) - In/Simulated ECUs/DrivekitCAN/Drivekit/TX/PDUs/THROTTLE_REPORT/throttle_operator_override/ISignal Value ==
  Const_throttle_operator_override Value : Constant  Value=0  OutDataTypeStr=uint8
  _ISignal Value_ : BusCreator  Inputs=1
  ISignal Value : Outport
  wires:
  _ISignal Value_/1 -> ISignal Value/1  "ISignal Value"
  Const_throttle_operator_override Value/1 -> _ISignal Value_/1  "throttle_operator_override Value"

== system ASM_Traffic_V2X_Complete_Model_2/IO/I//O_Subsystem/Bus Configuration (1) - In/Simulated ECUs/DrivekitCAN/Drivekit/TX/PDUs/THROTTLE_REPORT/throttle_report_enabled/ISignal Value ==
  Const_throttle_report_enabled Value : Constant  Value=0  OutDataTypeStr=uint8
  _ISignal Value_ : BusCreator  Inputs=1
  ISignal Value : Outport
  wires:
  _ISignal Value_/1 -> ISignal Value/1  "ISignal Value"
  Const_throttle_report_enabled Value/1 -> _ISignal Value_/1  "throttle_report_enabled Value"

== system ASM_Traffic_V2X_Complete_Model_2/IO/I//O_Subsystem/Bus Configuration (1) - In/Simulated ECUs/DrivekitCAN/Drivekit/TX/PDUs/THROTTLE_REPORT/throttle_report_magic/ISignal Value ==
  Const_throttle_report_magic Value : Constant  Value=0  OutDataTypeStr=uint16
  _ISignal Value_ : BusCreator  Inputs=1
  ISignal Value : Outport
  wires:
  _ISignal Value_/1 -> ISignal Value/1  "ISignal Value"
  Const_throttle_report_magic Value/1 -> _ISignal Value_/1  "throttle_report_magic Value"

== system ASM_Traffic_V2X_Complete_Model_2/IO/I//O_Subsystem/Bus Configuration (1) - In/Simulated ECUs/DrivekitCAN/Drivekit/TX/PDUs/WHL_SPD11/PDU Features/PDU Cyclic Timing Control ==
  Const_WHL_SPD11 Timing Control Offset : Constant  Value=0.02  OutDataTypeStr=double
  Const_WHL_SPD11 Timing Control Period : Constant  Value=0.02  OutDataTypeStr=double
  _PDU Cyclic Timing Control_ : BusCreator  Inputs=2
  PDU Cyclic Timing Control : Outport
  wires:
  _PDU Cyclic Timing Control_/1 -> PDU Cyclic Timing Control/1  "PDU Cyclic Timing Control"
  Const_WHL_SPD11 Timing Control Period/1 -> _PDU Cyclic Timing Control_/1  "WHL_SPD11 Timing Control Period"
  Const_WHL_SPD11 Timing Control Offset/1 -> _PDU Cyclic Timing Control_/2  "WHL_SPD11 Timing Control Offset"

== system ASM_Traffic_V2X_Complete_Model_2/IO/I//O_Subsystem/Bus Configuration (1) - In/Simulated ECUs/DrivekitCAN/Drivekit/TX/PDUs/WHL_SPD11/WHL_SPD_AliveCounter_LSB/ISignal Value ==
  Const_WHL_SPD_AliveCounter_LSB Value : Constant  Value=0  OutDataTypeStr=uint8
  _ISignal Value_ : BusCreator  Inputs=1
  ISignal Value : Outport
  wires:
  _ISignal Value_/1 -> ISignal Value/1  "ISignal Value"
  Const_WHL_SPD_AliveCounter_LSB Value/1 -> _ISignal Value_/1  "WHL_SPD_AliveCounter_LSB Value"

== system ASM_Traffic_V2X_Complete_Model_2/IO/I//O_Subsystem/Bus Configuration (1) - In/Simulated ECUs/DrivekitCAN/Drivekit/TX/PDUs/WHL_SPD11/WHL_SPD_AliveCounter_MSB/ISignal Value ==
  Const_WHL_SPD_AliveCounter_MSB Value : Constant  Value=0  OutDataTypeStr=uint8
  _ISignal Value_ : BusCreator  Inputs=1
  ISignal Value : Outport
  wires:
  _ISignal Value_/1 -> ISignal Value/1  "ISignal Value"
  Const_WHL_SPD_AliveCounter_MSB Value/1 -> _ISignal Value_/1  "WHL_SPD_AliveCounter_MSB Value"

== system ASM_Traffic_V2X_Complete_Model_2/IO/I//O_Subsystem/Bus Configuration (1) - In/Simulated ECUs/DrivekitCAN/Drivekit/TX/PDUs/WHL_SPD11/WHL_SPD_Checksum_LSB/ISignal Value ==
  Const_WHL_SPD_Checksum_LSB Value : Constant  Value=0  OutDataTypeStr=uint8
  _ISignal Value_ : BusCreator  Inputs=1
  ISignal Value : Outport
  wires:
  _ISignal Value_/1 -> ISignal Value/1  "ISignal Value"
  Const_WHL_SPD_Checksum_LSB Value/1 -> _ISignal Value_/1  "WHL_SPD_Checksum_LSB Value"

== system ASM_Traffic_V2X_Complete_Model_2/IO/I//O_Subsystem/Bus Configuration (1) - In/Simulated ECUs/DrivekitCAN/Drivekit/TX/PDUs/WHL_SPD11/WHL_SPD_Checksum_MSB/ISignal Value ==
  Const_WHL_SPD_Checksum_MSB Value : Constant  Value=0  OutDataTypeStr=uint8
  _ISignal Value_ : BusCreator  Inputs=1
  ISignal Value : Outport
  wires:
  _ISignal Value_/1 -> ISignal Value/1  "ISignal Value"
  Const_WHL_SPD_Checksum_MSB Value/1 -> _ISignal Value_/1  "WHL_SPD_Checksum_MSB Value"

== system ASM_Traffic_V2X_Complete_Model_2/IO/I//O_Subsystem/Bus Configuration (1) - In/Simulated ECUs/DrivekitCAN/Drivekit/TX/PDUs/WHL_SPD11/WHL_SPD_FL/ISignal Value ==
  Input : Inport
  Const_WHL_SPD_FL Value : Constant  Value=0  OutDataTypeStr=double
  Terminator : Terminator
  _ISignal Value_ : BusCreator  Inputs=1
  ISignal Value : Outport
  wires:
  _ISignal Value_/1 -> ISignal Value/1  "ISignal Value"
  Const_WHL_SPD_FL Value/1 -> Terminator/1  "WHL_SPD_FL Value"
  Input/1 -> _ISignal Value_/1  "WHL_SPD_FL Value"

== system ASM_Traffic_V2X_Complete_Model_2/IO/I//O_Subsystem/Bus Configuration (1) - In/Simulated ECUs/DrivekitCAN/Drivekit/TX/PDUs/WHL_SPD11/WHL_SPD_FR/ISignal Value ==
  Input : Inport
  Const_WHL_SPD_FR Value : Constant  Value=0  OutDataTypeStr=double
  Terminator : Terminator
  _ISignal Value_ : BusCreator  Inputs=1
  ISignal Value : Outport
  wires:
  _ISignal Value_/1 -> ISignal Value/1  "ISignal Value"
  Const_WHL_SPD_FR Value/1 -> Terminator/1  "WHL_SPD_FR Value"
  Input/1 -> _ISignal Value_/1  "WHL_SPD_FR Value"

== system ASM_Traffic_V2X_Complete_Model_2/IO/I//O_Subsystem/Bus Configuration (1) - In/Simulated ECUs/DrivekitCAN/Drivekit/TX/PDUs/WHL_SPD11/WHL_SPD_RL/ISignal Value ==
  Input : Inport
  Const_WHL_SPD_RL Value : Constant  Value=0  OutDataTypeStr=double
  Terminator : Terminator
  _ISignal Value_ : BusCreator  Inputs=1
  ISignal Value : Outport
  wires:
  _ISignal Value_/1 -> ISignal Value/1  "ISignal Value"
  Const_WHL_SPD_RL Value/1 -> Terminator/1  "WHL_SPD_RL Value"
  Input/1 -> _ISignal Value_/1  "WHL_SPD_RL Value"

== system ASM_Traffic_V2X_Complete_Model_2/IO/I//O_Subsystem/Bus Configuration (1) - In/Simulated ECUs/DrivekitCAN/Drivekit/TX/PDUs/WHL_SPD11/WHL_SPD_RR/ISignal Value ==
  Input : Inport
  Const_WHL_SPD_RR Value : Constant  Value=0  OutDataTypeStr=double
  Terminator : Terminator
  _ISignal Value_ : BusCreator  Inputs=1
  ISignal Value : Outport
  wires:
  _ISignal Value_/1 -> ISignal Value/1  "ISignal Value"
  Const_WHL_SPD_RR Value/1 -> Terminator/1  "WHL_SPD_RR Value"
  Input/1 -> _ISignal Value_/1  "WHL_SPD_RR Value"

== system ASM_Traffic_V2X_Complete_Model_2/IO/I//O_Subsystem/Bus Configuration (1) - Out/Simulated ECUs/DrivekitCAN/Drivekit/RX/PDUs/BRAKE_COMMAND/brake_command_magic/ISignal Value ==
  ISignal Value : Inport
  Term_brake_command_magic Value : Terminator
  _ISignal Value_ : BusSelector  OutputSignals=brake_command_magic Value
  wires:
  ISignal Value/1 -> _ISignal Value_/1  "ISignal Value"
  _ISignal Value_/1 -> Term_brake_command_magic Value/1  "<brake_command_magic Value>"

== system ASM_Traffic_V2X_Complete_Model_2/IO/I//O_Subsystem/Bus Configuration (1) - Out/Simulated ECUs/DrivekitCAN/Drivekit/RX/PDUs/BRAKE_COMMAND/brake_pedal_command/ISignal Value ==
  ISignal Value : Inport
  Term_brake_pedal_command Value : Terminator
  _ISignal Value_ : BusSelector  OutputSignals=brake_pedal_command Value
  wires:
  ISignal Value/1 -> _ISignal Value_/1  "ISignal Value"
  _ISignal Value_/1 -> Term_brake_pedal_command Value/1  "<brake_pedal_command Value>"

== system ASM_Traffic_V2X_Complete_Model_2/IO/I//O_Subsystem/Bus Configuration (1) - Out/Simulated ECUs/DrivekitCAN/Drivekit/RX/PDUs/BRAKE_DISABLE/brake_disable_magic/ISignal Value ==
  ISignal Value : Inport
  Term_brake_disable_magic Value : Terminator
  _ISignal Value_ : BusSelector  OutputSignals=brake_disable_magic Value
  wires:
  ISignal Value/1 -> _ISignal Value_/1  "ISignal Value"
  _ISignal Value_/1 -> Term_brake_disable_magic Value/1  "<brake_disable_magic Value>"

== system ASM_Traffic_V2X_Complete_Model_2/IO/I//O_Subsystem/Bus Configuration (1) - Out/Simulated ECUs/DrivekitCAN/Drivekit/RX/PDUs/BRAKE_ENABLE/brake_enable_magic/ISignal Value ==
  ISignal Value : Inport
  Term_brake_enable_magic Value : Terminator
  _ISignal Value_ : BusSelector  OutputSignals=brake_enable_magic Value
  wires:
  ISignal Value/1 -> _ISignal Value_/1  "ISignal Value"
  _ISignal Value_/1 -> Term_brake_enable_magic Value/1  "<brake_enable_magic Value>"

== system ASM_Traffic_V2X_Complete_Model_2/IO/I//O_Subsystem/Bus Configuration (1) - Out/Simulated ECUs/DrivekitCAN/Drivekit/RX/PDUs/CHASSIS_CONTROL_COMMAND/front_wipers/ISignal Value ==
  ISignal Value : Inport
  Term_front_wipers Value : Terminator
  _ISignal Value_ : BusSelector  OutputSignals=front_wipers Value
  wires:
  ISignal Value/1 -> _ISignal Value_/1  "ISignal Value"
  _ISignal Value_/1 -> Term_front_wipers Value/1  "<front_wipers Value>"

== system ASM_Traffic_V2X_Complete_Model_2/IO/I//O_Subsystem/Bus Configuration (1) - Out/Simulated ECUs/DrivekitCAN/Drivekit/RX/PDUs/CHASSIS_CONTROL_COMMAND/headlamps/ISignal Value ==
  ISignal Value : Inport
  Term_headlamps Value : Terminator
  _ISignal Value_ : BusSelector  OutputSignals=headlamps Value
  wires:
  ISignal Value/1 -> _ISignal Value_/1  "ISignal Value"
  _ISignal Value_/1 -> Term_headlamps Value/1  "<headlamps Value>"

== system ASM_Traffic_V2X_Complete_Model_2/IO/I//O_Subsystem/Bus Configuration (1) - Out/Simulated ECUs/DrivekitCAN/Drivekit/RX/PDUs/CHASSIS_CONTROL_COMMAND/horn/ISignal Value ==
  ISignal Value : Inport
  Term_horn Value : Terminator
  _ISignal Value_ : BusSelector  OutputSignals=horn Value
  wires:
  ISignal Value/1 -> _ISignal Value_/1  "ISignal Value"
  _ISignal Value_/1 -> Term_horn Value/1  "<horn Value>"
